simulink model "SerialMonitor_withPRBS"  (R2016b)
settings: Solver=FixedStepDiscrete  StartTime=0.0  StopTime=inf  FixedStep=.01  RelTol=1e-3  EnableMultiTasking=on
StartFcn:
  | s_2 = serial(Port,'BaudRate',115200,'FlowControl','none','Parity','none','DataBits',8,'StopBits',1,'Timeout',2);
  | s_2.InputBufferSize=1024*5; s_2.OutputBufferSize=1024*5;
  | s_2.Terminator='CR';
  | 
  | fopen(s_2);
StopFcn:
  | fclose(s_2);
undefined symbols (not defined in the file or in its folder): serialRead, serialWriteLightBox
libraries: simulink x36, sldrtlib x1
settings Model: Creator=EliteBook 8470p  LastModifiedBy=rsjoshi1
settings DataIOCC: LimitDataPoints=on  SaveFormat=Array
settings OptimizationCC: LifeSpan=inf
settings DebuggingCC: SolverPrmCheckMsg=warning  SFUnexpectedBacktrackingDiag=warning  SFNoUnconditionalDefaultTransitionDiag=warning  SFExecutionAtInitializationDiag=none
settings HardwareCC: ProdBitPerPointer=32  ProdBitPerSizeT=32  ProdBitPerPtrDiffT=32  ProdLargestAtomicFloat=None  ProdIntDivRoundTo=Undefined  ProdEndianess=Unspecified  ProdWordSize=32  ProdHWDeviceType=32-bit Generic
settings ModelReferenceCC: PropagateSignalLabelsOutOfModel=off
settings GRTTargetCC: TargetLangStandard=C89/C90 (ANSI)  GeneratePreprocessorConditionals=Disable all
settings ConfigComp: CovMetricSettings=dw  CovHtmlReporting=on  CovSaveCumulativeToWorkspaceVar=on  CovSaveSingleToWorkspaceVar=on  CovExternalEMLEnable=off  CovSFcnEnable=off

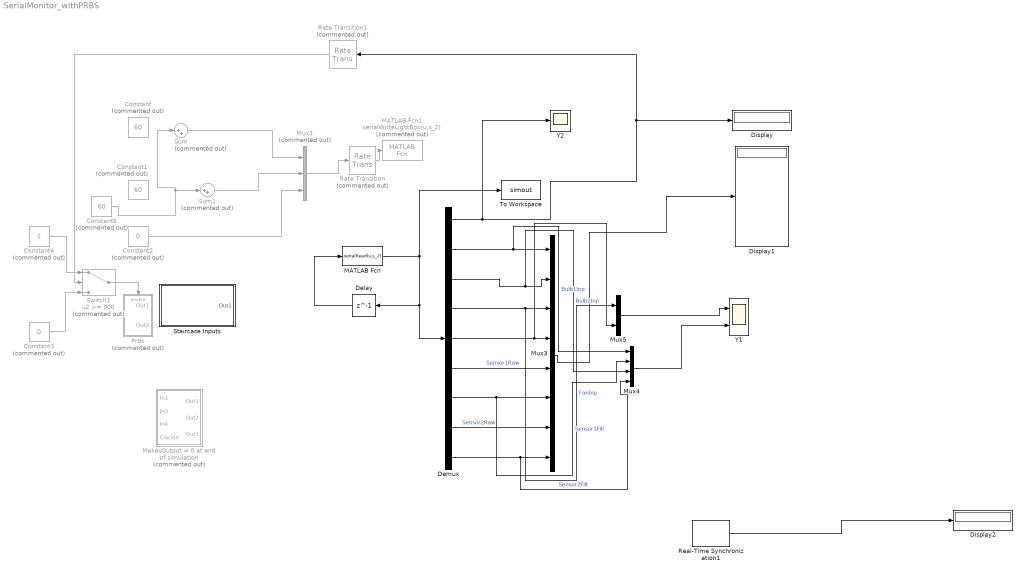
== system SerialMonitor_withPRBS ==
  Constant : Constant  Commented=on  Value=60  OutDataTypeStr=double  SampleTime=0.1
  Constant1 : Constant  Commented=on  Value=60  OutDataTypeStr=double  SampleTime=0.1
  Constant2 : Constant  Commented=on  Value=0  OutDataTypeStr=double  SampleTime=0.1
  Constant3 : Constant  Commented=on  Value=0  SampleTime=0.1
  Constant4 : Constant  Commented=on  SampleTime=0.1
  Constant6 : Constant  Commented=on  Value=60  OutDataTypeStr=double  SampleTime=0.1
  Delay : Delay  DelayLength=1  InitialCondition=0  SampleTime=1
  Demux : Demux  Outputs=9
  Display : Display
  Display1 : Display
  Display2 : Display
  MATLAB Fcn : MATLABFcn  MATLABFcn=serialRead(u,s_2)  OutputDimensions=9
  MATLAB Fcn1 : MATLABFcn  Commented=on  MATLABFcn=serialWriteLightBox(u,s_2)  OutputDimensions=0
  MakesOutput = 0 at end of simulation : Subsystem  Commented=on
  Mux1 : Mux  Commented=on  Inputs=3
  Mux3 : Mux  Inputs=8
  Mux4 : Mux
  Mux5 : Mux  Inputs=2
  Prbs : Subsystem  Commented=on
  Rate Transition : RateTransition  Commented=on  Deterministic=off  OutPortSampleTime=1
  Rate Transition1 : RateTransition  Commented=on  OutPortSampleTime=0.1
  Real-Time Synchronization1 : sldrtlib/Real-Time Synchronization  SampleTime=0.1  MaxMissedTicks=5000  ShowMissedTicks=on  YieldWhenWaiting=off
  Staircase Inputs : Subsystem
  Sum : Sum  Commented=on  Inputs=|++
  Sum1 : Sum  Commented=on  Inputs=|++
  Switch1 : Switch  Commented=on  Threshold=900  SampleTime=0.1
  To Workspace : ToWorkspace  VariableName=simout  SaveFormat=Structure With Time  SampleTime=-1
  Y1 : Scope  NumInputPorts=2
  Y2 : Scope
  wires:
  Delay/1 -> MATLAB Fcn/1
  MATLAB Fcn/1 -> Demux/1, Delay/1, To Workspace/1
  Demux/2 -> Mux4/1, Mux3/1  "Bulb1Inp"
  Demux/3 -> Mux4/3, Mux3/2  "Bulb2Inp"
  Demux/4 -> Mux5/1, Mux3/3  "FanInp"
  Demux/5 -> Mux5/2, Mux3/4
  Demux/6 -> Mux3/5  "Sensor1Raw"
  Demux/7 -> Mux4/2, Mux3/6  "Sensor1Filt"
  Demux/8 -> Mux3/7  "Sensor2Raw"
  Mux1/1 -> Rate Transition/1
  Rate Transition/1 -> MATLAB Fcn1/1
  Real-Time Synchronization1/1 -> Display2/1
  Mux3/1 -> Display1/1
  Constant3/1 -> Switch1/3
  Constant4/1 -> Switch1/1
  Switch1/1 -> Prbs/Enable
  Demux/1 -> Y2/1, Rate Transition1/1, Display/1
  Sum1/1 -> Mux1/2
  Sum/1 -> Mux1/1
  Constant2/1 -> Mux1/3
  Rate Transition1/1 -> Switch1/2
  Demux/9 -> Mux4/4, Mux3/8  "Sensor2Filt"
  Mux4/1 -> Y1/2
  Mux5/1 -> Y1/1
  Constant6/1 -> Sum/1, Sum1/1

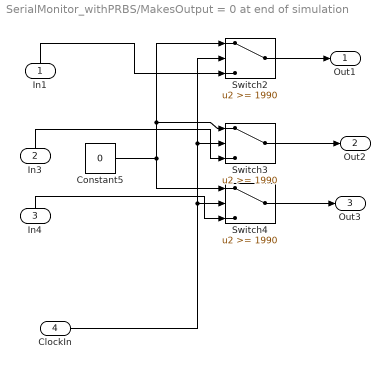
== system SerialMonitor_withPRBS/MakesOutput = 0 at end of simulation ==
  In1 : Inport
  In3 : Inport  Port=2
  In4 : Inport  Port=3
  ClockIn : Inport  Port=4
  Constant5 : Constant  Value=0  SampleTime=0.1
  Switch2 : Switch  Threshold=1990  SampleTime=0.1
  Switch3 : Switch  Threshold=1990  SampleTime=0.1
  Switch4 : Switch  Threshold=1990  SampleTime=0.1
  Out1 : Outport
  Out2 : Outport  Port=2
  Out3 : Outport  Port=3
  wires:
  Switch2/1 -> Out1/1
  ClockIn/1 -> Switch2/2, Switch3/2, Switch4/2
  In1/1 -> Switch2/3
  Switch3/1 -> Out2/1
  In4/1 -> Switch4/3
  Switch4/1 -> Out3/1
  In3/1 -> Switch3/3
  Constant5/1 -> Switch4/1, Switch2/1, Switch3/1

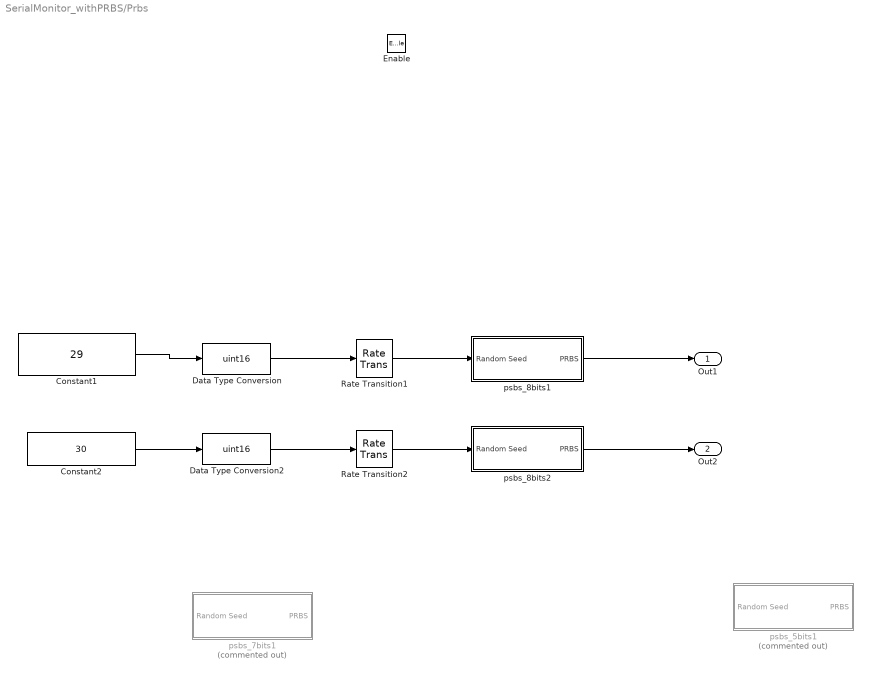
== system SerialMonitor_withPRBS/Prbs ==
  Enable : EnablePort
  Constant1 : Constant  Value=29  OutDataTypeStr=double  SampleTime=0.1
  Constant2 : Constant  Value=30  OutDataTypeStr=double  SampleTime=0.1
  Data Type Conversion : DataTypeConversion  OutDataTypeStr=uint16
  Data Type Conversion2 : DataTypeConversion  OutDataTypeStr=uint16
  Rate Transition1 : RateTransition  OutPortSampleTime=0.1
  Rate Transition2 : RateTransition  OutPortSampleTime=0.1
  psbs_5bits1 : Subsystem  Commented=on  mask(PRBS with 8 shift registers){T=0.1, Tsw=60, Lz=10, Lv=300, Nc=1}
      mask prompts: T "Sample Time (s)"; Tsw "Time to switch (s)"; Lz "Leading Zeros (s)"; Lv "Switching Levels"; Nc "Number of Cycles"
      mask help:
      | Creates a PRBS signal using 6 shift registers.
      |     *Time to switch (Tsw) must be an integer multiple of Sample Time (T).
      |     *Leading zeros specify how long the PRBS will be zero, in seconds, before the levels begin shifting.
      |     *Level is the amplitude of the desired PRBS signal. Both + and - levels are equal
      |     *Number of cycles determines the number of full cycles generated. Each cycle is (2^6-1)*Tsw seconds long
  psbs_7bits1 : Subsystem  Commented=on  mask(PRBS with 8 shift registers){T=0.1, Tsw=60, Lz=10, Lv=300, Nc=1}
      mask prompts: T "Sample Time (s)"; Tsw "Time to switch (s)"; Lz "Leading Zeros (s)"; Lv "Switching Levels"; Nc "Number of Cycles"
      mask help:
      | Creates a PRBS signal using 7 shift registers.
      |     *Time to switch (Tsw) must be an integer multiple of Sample Time (T).
      |     *Leading zeros specify how long the PRBS will be zero, in seconds, before the levels begin shifting.
      |     *Level is the amplitude of the desired PRBS signal. Both + and - levels are equal
      |     *Number of cycles determines the number of full cycles generated. Each cycle is (2^7-1)*Tsw seconds long
  psbs_8bits1 : Subsystem  mask(PRBS with 8 shift registers){T=0.1, Tsw=20, Lz=50, Lv=300, Nc=1}
      mask prompts: T "Sample Time (s)"; Tsw "Time to switch (s)"; Lz "Leading Zeros (s)"; Lv "Switching Levels"; Nc "Number of Cycles"
      mask help:
      | Creates a PRBS signal using 8 shift registers.
      |     *Time to switch (Tsw) must be an integer multiple of Sample Time (T).
      |     *Leading zeros specify how long the PRBS will be zero, in seconds, before the levels begin shifting.
      |     *Level is the amplitude of the desired PRBS signal. Both + and - levels are equal
      |     *Number of cycles determines the number of full cycles generated. Each cycle is (2^8-1)*Tsw seconds long
  psbs_8bits2 : Subsystem  mask(PRBS with 8 shift registers){T=0.1, Tsw=20, Lz=50, Lv=300, Nc=1}
      mask prompts: T "Sample Time (s)"; Tsw "Time to switch (s)"; Lz "Leading Zeros (s)"; Lv "Switching Levels"; Nc "Number of Cycles"
      mask help:
      | Creates a PRBS signal using 8 shift registers.
      |     *Time to switch (Tsw) must be an integer multiple of Sample Time (T).
      |     *Leading zeros specify how long the PRBS will be zero, in seconds, before the levels begin shifting.
      |     *Level is the amplitude of the desired PRBS signal. Both + and - levels are equal
      |     *Number of cycles determines the number of full cycles generated. Each cycle is (2^8-1)*Tsw seconds long
  Out1 : Outport
  Out2 : Outport  Port=2
  wires:
  Constant1/1 -> Data Type Conversion/1
  Data Type Conversion/1 -> Rate Transition1/1
  psbs_8bits1/1(PRBS) -> Out1/1
  Rate Transition1/1 -> psbs_8bits1/1(Random Seed)
  psbs_8bits2/1(PRBS) -> Out2/1
  Rate Transition2/1 -> psbs_8bits2/1(Random Seed)
  Constant2/1 -> Data Type Conversion2/1
  Data Type Conversion2/1 -> Rate Transition2/1

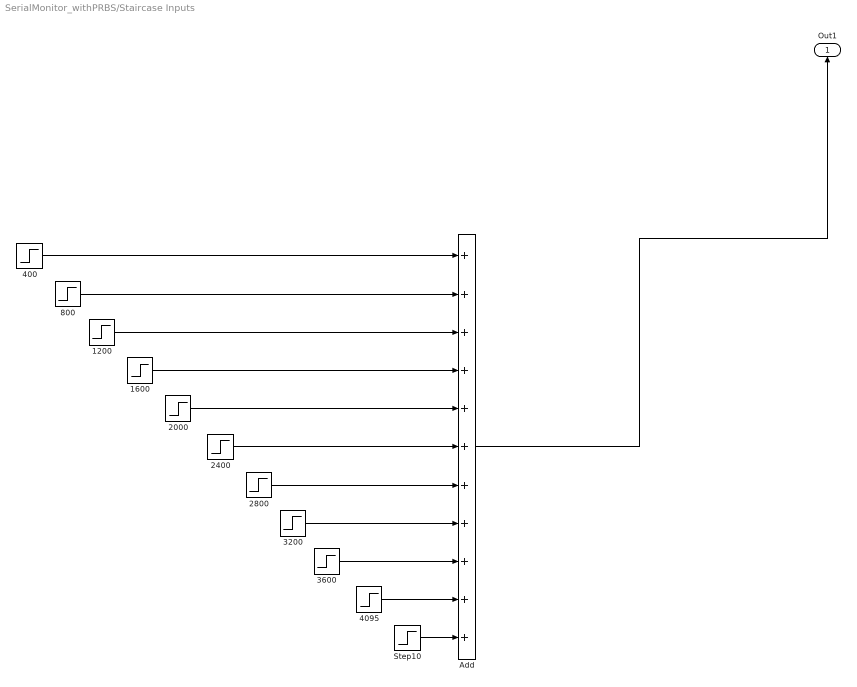
== system SerialMonitor_withPRBS/Staircase Inputs ==
  1200 : Step  Time=70*60  After=400  SampleTime=0.1
  1600 : Step  Time=100*60  After=400  SampleTime=0.1
  2000 : Step  Time=130*60  After=400  SampleTime=0.1
  2400 : Step  Time=160*60  After=400  SampleTime=0.1
  2800 : Step  Time=190*60  After=400  SampleTime=0.1
  3200 : Step  Time=220*60  After=400  SampleTime=0.1
  3600 : Step  Time=250*60  After=400  SampleTime=0.1
  400 : Step  Time=100  After=400  SampleTime=0.1
  4095 : Step  Time=280*60  After=495  SampleTime=0.1
  800 : Step  Time=40*60  After=400  SampleTime=0.1
  Add : Sum  Inputs=+++++++++++
  Step10 : Step  Time=310*60  After=-4095  SampleTime=0.1
  Out1 : Outport
  wires:
  Step10/1 -> Add/11
  3600/1 -> Add/9
  2400/1 -> Add/6
  1200/1 -> Add/3
  3200/1 -> Add/8
  800/1 -> Add/2
  2000/1 -> Add/5
  400/1 -> Add/1
  2800/1 -> Add/7
  1600/1 -> Add/4
  4095/1 -> Add/10
  Add/1 -> Out1/1

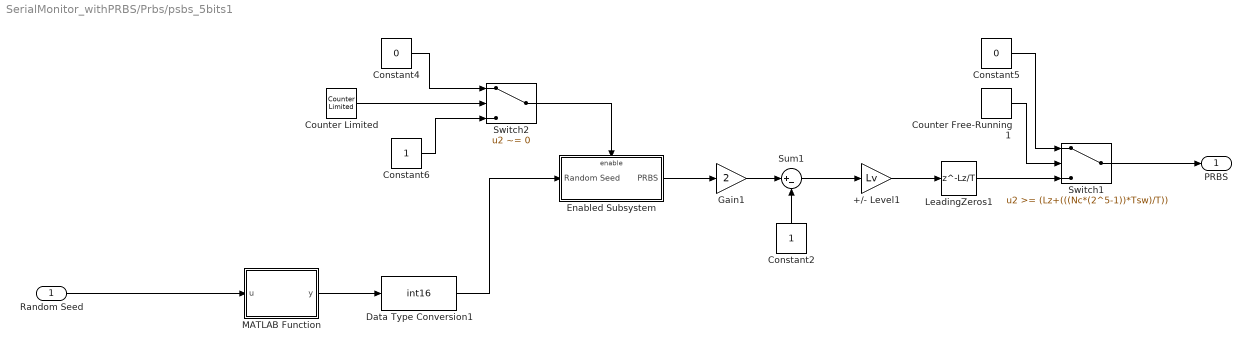
== system SerialMonitor_withPRBS/Prbs/psbs_5bits1 ==
  Random Seed : Inport  OutDataTypeStr=uint16
  +/- Level1 : Gain  Gain=Lv  SampleTime=T
  Constant2 : Constant  SampleTime=T
  Constant4 : Constant  Value=0  SampleTime=T
  Constant5 : Constant  Value=0  SampleTime=T
  Constant6 : Constant  SampleTime=T
  Counter Free-Running1 : simulink/Sources/Counter Free-Running  NumBits=32  tsamp=T
  Counter Limited : simulink/Sources/Counter Limited  uplimit=Tsw/T-1  tsamp=T
  Data Type Conversion1 : DataTypeConversion  OutDataTypeStr=int16
  Enabled Subsystem : Subsystem  TreatAsAtomicUnit=on
  Gain1 : Gain  Gain=2  SampleTime=T
  LeadingZeros1 : Delay  DelayLength=Lz/T  InitialCondition=0  SampleTime=T
  MATLAB Function : MATLAB Function  TreatAsAtomicUnit=on
  Sum1 : Sum  Inputs=|+-  SampleTime=T
  Switch1 : Switch  Threshold=(Lz+(((Nc*(2^5-1))*Tsw)/T))  SampleTime=T
  Switch2 : Switch  Criteria=u2 ~= 0  Threshold=Tsw/T  SampleTime=T
  PRBS : Outport
  wires:
  Counter Limited/1 -> Switch2/2
  Switch2/1 -> Enabled Subsystem/Enable
  Constant4/1 -> Switch2/1
  Constant6/1 -> Switch2/3
  Data Type Conversion1/1 -> Enabled Subsystem/1(Random Seed)
  Enabled Subsystem/1(PRBS) -> Gain1/1
  Sum1/1 -> +/- Level1/1
  Gain1/1 -> Sum1/1
  Constant2/1 -> Sum1/2
  Counter Free-Running1/1 -> Switch1/2
  +/- Level1/1 -> LeadingZeros1/1
  Constant5/1 -> Switch1/1
  LeadingZeros1/1 -> Switch1/3
  MATLAB Function/1(y) -> Data Type Conversion1/1
  Random Seed/1 -> MATLAB Function/1(u)
  Switch1/1 -> PRBS/1

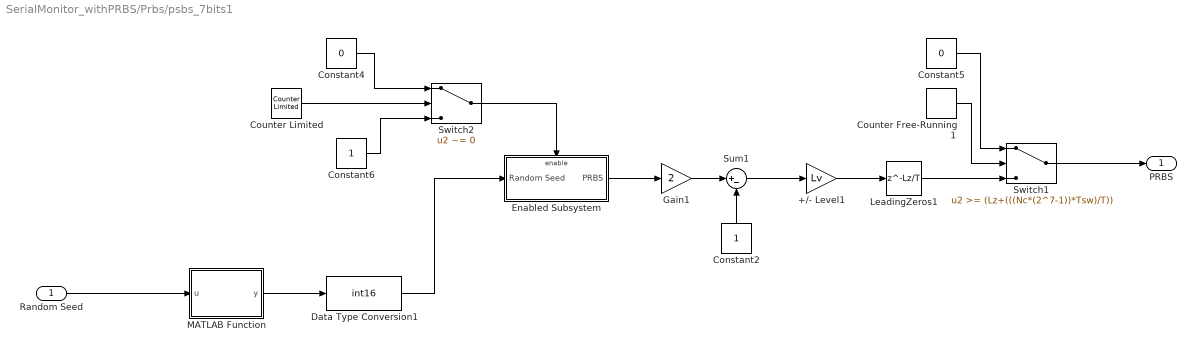
== system SerialMonitor_withPRBS/Prbs/psbs_7bits1 ==
  Random Seed : Inport  OutDataTypeStr=uint16
  +/- Level1 : Gain  Gain=Lv  SampleTime=T
  Constant2 : Constant  SampleTime=T
  Constant4 : Constant  Value=0  SampleTime=T
  Constant5 : Constant  Value=0  SampleTime=T
  Constant6 : Constant  SampleTime=T
  Counter Free-Running1 : simulink/Sources/Counter Free-Running  NumBits=32  tsamp=T
  Counter Limited : simulink/Sources/Counter Limited  uplimit=Tsw/T-1  tsamp=T
  Data Type Conversion1 : DataTypeConversion  OutDataTypeStr=int16
  Enabled Subsystem : Subsystem  TreatAsAtomicUnit=on
  Gain1 : Gain  Gain=2  SampleTime=T
  LeadingZeros1 : Delay  DelayLength=Lz/T  InitialCondition=0  SampleTime=T
  MATLAB Function : MATLAB Function  TreatAsAtomicUnit=on
  Sum1 : Sum  Inputs=|+-  SampleTime=T
  Switch1 : Switch  Threshold=(Lz+(((Nc*(2^7-1))*Tsw)/T))  SampleTime=T
  Switch2 : Switch  Criteria=u2 ~= 0  Threshold=Tsw/T  SampleTime=T
  PRBS : Outport
  wires:
  Switch1/1 -> PRBS/1
  Random Seed/1 -> MATLAB Function/1(u)
  MATLAB Function/1(y) -> Data Type Conversion1/1
  LeadingZeros1/1 -> Switch1/3
  Constant5/1 -> Switch1/1
  +/- Level1/1 -> LeadingZeros1/1
  Counter Free-Running1/1 -> Switch1/2
  Constant2/1 -> Sum1/2
  Gain1/1 -> Sum1/1
  Sum1/1 -> +/- Level1/1
  Enabled Subsystem/1(PRBS) -> Gain1/1
  Data Type Conversion1/1 -> Enabled Subsystem/1(Random Seed)
  Constant6/1 -> Switch2/3
  Constant4/1 -> Switch2/1
  Switch2/1 -> Enabled Subsystem/Enable
  Counter Limited/1 -> Switch2/2

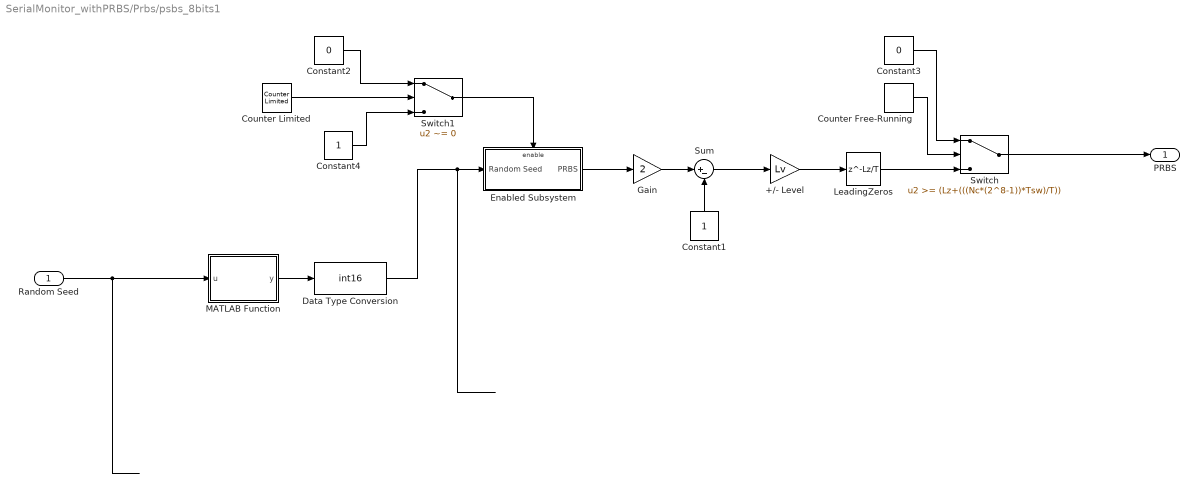
== system SerialMonitor_withPRBS/Prbs/psbs_8bits1 ==
  Random Seed : Inport  OutDataTypeStr=uint16  SampleTime=0.1
  +/- Level : Gain  Gain=Lv  SampleTime=T
  Constant1 : Constant  SampleTime=T
  Constant2 : Constant  Value=0  SampleTime=T
  Constant3 : Constant  Value=0  SampleTime=T
  Constant4 : Constant  SampleTime=T
  Counter Free-Running : simulink/Sources/Counter Free-Running  NumBits=32  tsamp=T
  Counter Limited : simulink/Sources/Counter Limited  uplimit=Tsw/T-1  tsamp=T
  Data Type Conversion : DataTypeConversion  OutDataTypeStr=int16
  Enabled Subsystem : Subsystem  TreatAsAtomicUnit=on
  Gain : Gain  Gain=2  SampleTime=T
  LeadingZeros : Delay  DelayLength=Lz/T  InitialCondition=0  SampleTime=T
  MATLAB Function : MATLAB Function  TreatAsAtomicUnit=on
  Sum : Sum  Inputs=|+-  SampleTime=T
  Switch : Switch  Threshold=(Lz+(((Nc*(2^8-1))*Tsw)/T))  SampleTime=T
  Switch1 : Switch  Criteria=u2 ~= 0  Threshold=Tsw/T  SampleTime=T
  PRBS : Outport
  wires:
  Random Seed/1 -> MATLAB Function/1(u)
  Counter Limited/1 -> Switch1/2
  Switch1/1 -> Enabled Subsystem/Enable
  Constant2/1 -> Switch1/1
  Constant4/1 -> Switch1/3
  Data Type Conversion/1 -> Enabled Subsystem/1(Random Seed)
  Enabled Subsystem/1(PRBS) -> Gain/1
  Sum/1 -> +/- Level/1
  Gain/1 -> Sum/1
  Constant1/1 -> Sum/2
  Counter Free-Running/1 -> Switch/2
  +/- Level/1 -> LeadingZeros/1
  Constant3/1 -> Switch/1
  LeadingZeros/1 -> Switch/3
  MATLAB Function/1(y) -> Data Type Conversion/1
  Switch/1 -> PRBS/1

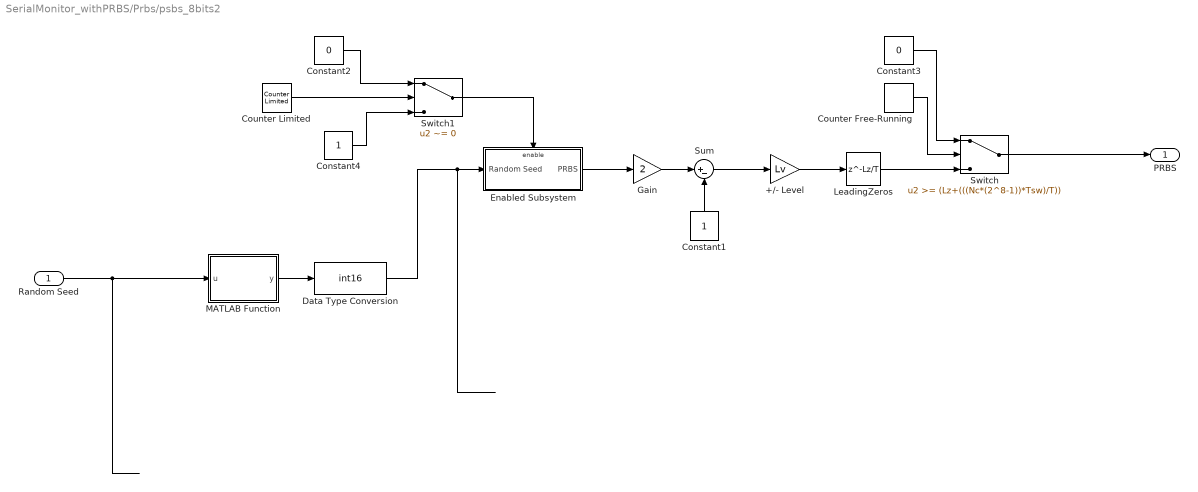
== system SerialMonitor_withPRBS/Prbs/psbs_8bits2 ==
  Random Seed : Inport  OutDataTypeStr=uint16  SampleTime=0.1
  +/- Level : Gain  Gain=Lv  SampleTime=T
  Constant1 : Constant  SampleTime=T
  Constant2 : Constant  Value=0  SampleTime=T
  Constant3 : Constant  Value=0  SampleTime=T
  Constant4 : Constant  SampleTime=T
  Counter Free-Running : simulink/Sources/Counter Free-Running  NumBits=32  tsamp=T
  Counter Limited : simulink/Sources/Counter Limited  uplimit=Tsw/T-1  tsamp=T
  Data Type Conversion : DataTypeConversion  OutDataTypeStr=int16
  Enabled Subsystem : Subsystem  TreatAsAtomicUnit=on
  Gain : Gain  Gain=2  SampleTime=T
  LeadingZeros : Delay  DelayLength=Lz/T  InitialCondition=0  SampleTime=T
  MATLAB Function : MATLAB Function  TreatAsAtomicUnit=on
  Sum : Sum  Inputs=|+-  SampleTime=T
  Switch : Switch  Threshold=(Lz+(((Nc*(2^8-1))*Tsw)/T))  SampleTime=T
  Switch1 : Switch  Criteria=u2 ~= 0  Threshold=Tsw/T  SampleTime=T
  PRBS : Outport
  wires:
  Switch/1 -> PRBS/1
  MATLAB Function/1(y) -> Data Type Conversion/1
  LeadingZeros/1 -> Switch/3
  Constant3/1 -> Switch/1
  +/- Level/1 -> LeadingZeros/1
  Counter Free-Running/1 -> Switch/2
  Constant1/1 -> Sum/2
  Gain/1 -> Sum/1
  Sum/1 -> +/- Level/1
  Enabled Subsystem/1(PRBS) -> Gain/1
  Data Type Conversion/1 -> Enabled Subsystem/1(Random Seed)
  Constant4/1 -> Switch1/3
  Constant2/1 -> Switch1/1
  Switch1/1 -> Enabled Subsystem/Enable
  Counter Limited/1 -> Switch1/2
  Random Seed/1 -> MATLAB Function/1(u)

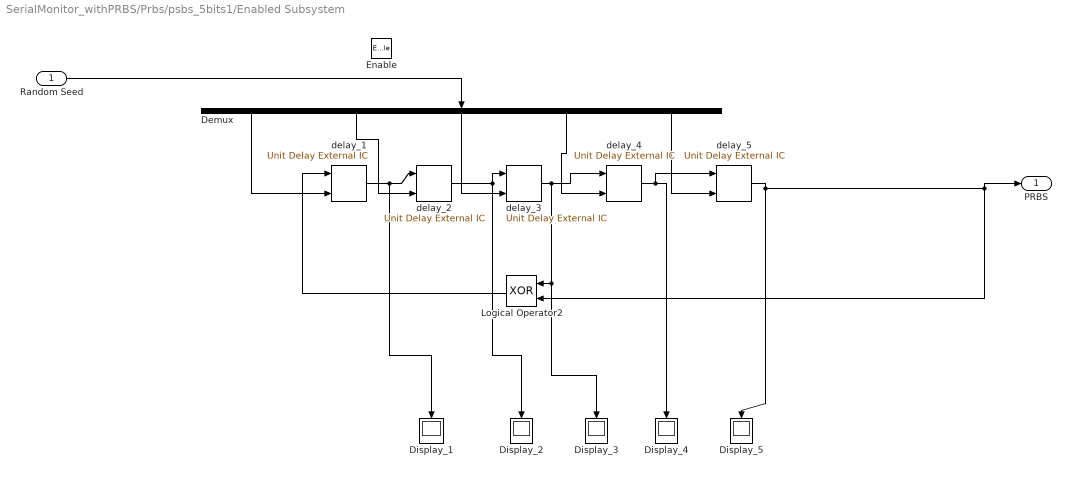
== system SerialMonitor_withPRBS/Prbs/psbs_5bits1/Enabled Subsystem ==
  Random Seed : Inport  OutDataTypeStr=int16
  Enable : EnablePort
  Demux : Demux  Outputs=5
  Display_{1..5} (5 alike) : Display
  Logical Operator2 : Logic  Operator=XOR  AllPortsSameDT=off  OutDataTypeStr=fixdt(1,16)  SampleTime=T
  delay_{1..5} (5 alike) : simulink/Additional Math & Discrete/Additional Discrete/Unit Delay External IC  tsamp=T
  PRBS : Outport
  wires:
  Random Seed/1 -> Demux/1
  delay_5/1 -> Logical Operator2/2, PRBS/1, Display_5/1
  Logical Operator2/1 -> delay_1/1
  Demux/1 -> delay_1/2
  Demux/2 -> delay_2/2
  Demux/3 -> delay_3/2
  Demux/4 -> delay_4/2
  Demux/5 -> delay_5/2
  delay_1/1 -> Display_1/1, delay_2/1
  delay_4/1 -> Display_4/1, delay_5/1
  delay_3/1 -> delay_4/1, Logical Operator2/1, Display_3/1
  delay_2/1 -> delay_3/1, Display_2/1

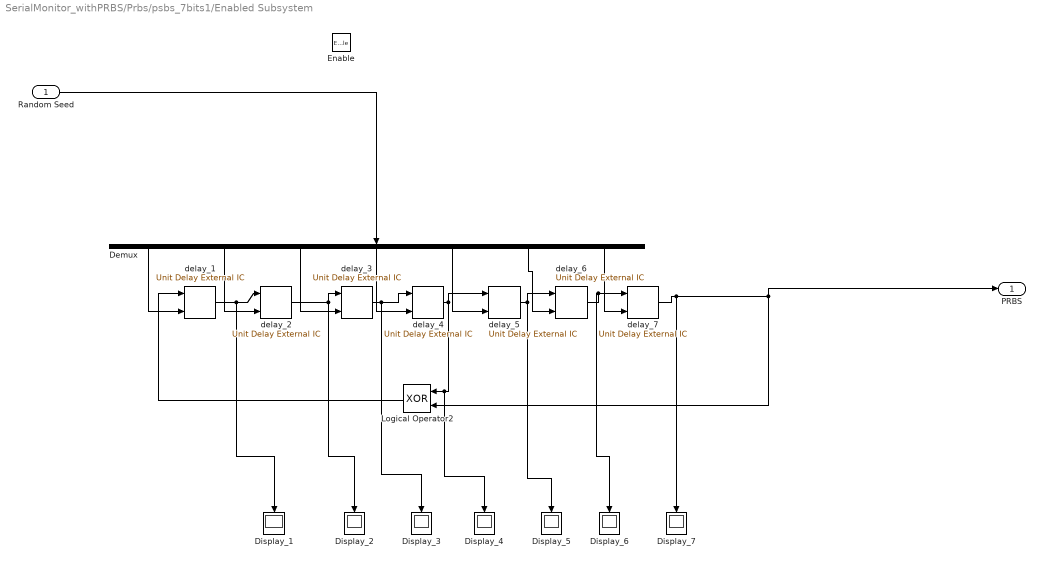
== system SerialMonitor_withPRBS/Prbs/psbs_7bits1/Enabled Subsystem ==
  Random Seed : Inport  OutDataTypeStr=int16
  Enable : EnablePort
  Demux : Demux  Outputs=7
  Display_{1..7} (7 alike) : Display
  Logical Operator2 : Logic  Operator=XOR  AllPortsSameDT=off  OutDataTypeStr=fixdt(1,16)  SampleTime=T
  delay_{1..7} (7 alike) : simulink/Additional Math & Discrete/Additional Discrete/Unit Delay External IC  tsamp=T
  PRBS : Outport
  wires:
  delay_7/1 -> Logical Operator2/2, PRBS/1, Display_7/1
  delay_5/1 -> Display_5/1, delay_6/1
  delay_6/1 -> Display_6/1, delay_7/1
  delay_2/1 -> Display_2/1, delay_3/1
  delay_3/1 -> Display_3/1, delay_4/1
  delay_4/1 -> Display_4/1, Logical Operator2/1, delay_5/1
  delay_1/1 -> delay_2/1, Display_1/1
  Demux/7 -> delay_7/2
  Demux/6 -> delay_6/2
  Demux/5 -> delay_5/2
  Demux/4 -> delay_4/2
  Demux/3 -> delay_3/2
  Demux/2 -> delay_2/2
  Demux/1 -> delay_1/2
  Random Seed/1 -> Demux/1
  Logical Operator2/1 -> delay_1/1

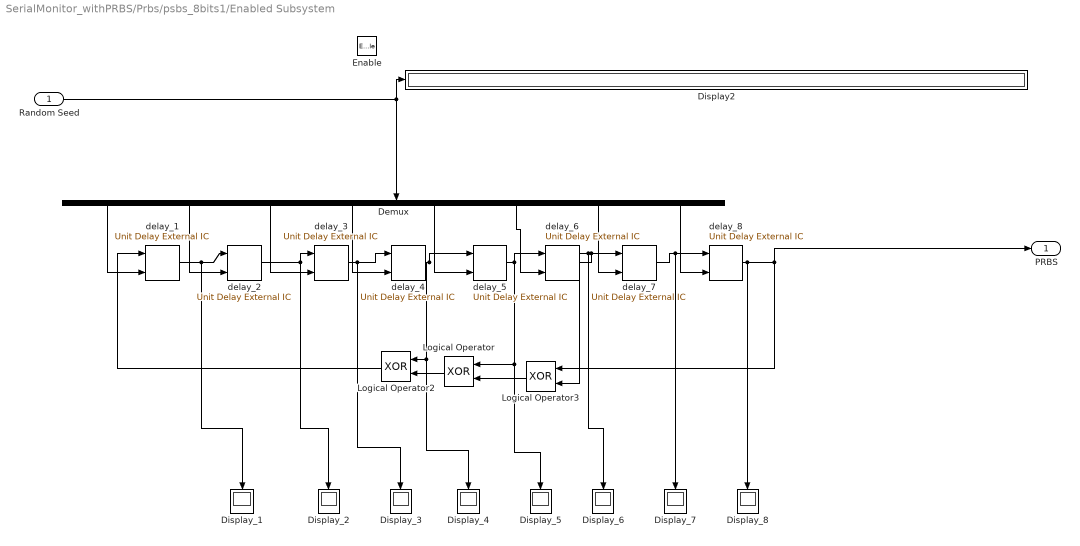
== system SerialMonitor_withPRBS/Prbs/psbs_8bits1/Enabled Subsystem ==
  Random Seed : Inport  OutDataTypeStr=int16
  Enable : EnablePort
  Demux : Demux  Outputs=8
  Display2 : Display
  Display_{1..8} (8 alike) : Display
  Logical Operator : Logic  Operator=XOR  AllPortsSameDT=off  OutDataTypeStr=fixdt(1,16)  SampleTime=T
  Logical Operator2 : Logic  Operator=XOR  AllPortsSameDT=off  OutDataTypeStr=fixdt(1,16)  SampleTime=T
  Logical Operator3 : Logic  Operator=XOR  AllPortsSameDT=off  OutDataTypeStr=fixdt(1,16)  SampleTime=T
  delay_{1..8} (8 alike) : simulink/Additional Math & Discrete/Additional Discrete/Unit Delay External IC  tsamp=T
  PRBS : Outport
  wires:
  delay_5/1 -> Display_5/1, Logical Operator/1, delay_6/1
  delay_6/1 -> Logical Operator3/2, Display_6/1, delay_7/1
  delay_2/1 -> Display_2/1, delay_3/1
  delay_3/1 -> Display_3/1, delay_4/1
  delay_4/1 -> Display_4/1, Logical Operator2/1, delay_5/1
  delay_1/1 -> delay_2/1, Display_1/1
  delay_7/1 -> Display_7/1, delay_8/1
  Logical Operator/1 -> Logical Operator2/2
  Logical Operator3/1 -> Logical Operator/2
  Random Seed/1 -> Display2/1, Demux/1
  Demux/8 -> delay_8/2
  Demux/7 -> delay_7/2
  Demux/6 -> delay_6/2
  Demux/5 -> delay_5/2
  Demux/4 -> delay_4/2
  Demux/3 -> delay_3/2
  Demux/2 -> delay_2/2
  Demux/1 -> delay_1/2
  Logical Operator2/1 -> delay_1/1
  delay_8/1 -> Logical Operator3/1, PRBS/1, Display_8/1

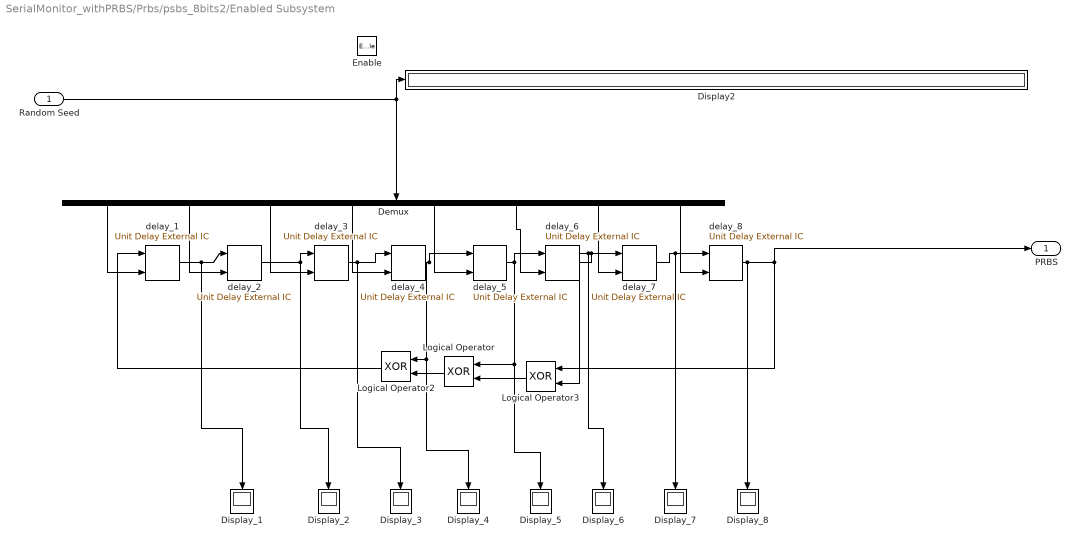
== system SerialMonitor_withPRBS/Prbs/psbs_8bits2/Enabled Subsystem ==
  Random Seed : Inport  OutDataTypeStr=int16
  Enable : EnablePort
  Demux : Demux  Outputs=8
  Display2 : Display
  Display_{1..8} (8 alike) : Display
  Logical Operator : Logic  Operator=XOR  AllPortsSameDT=off  OutDataTypeStr=fixdt(1,16)  SampleTime=T
  Logical Operator2 : Logic  Operator=XOR  AllPortsSameDT=off  OutDataTypeStr=fixdt(1,16)  SampleTime=T
  Logical Operator3 : Logic  Operator=XOR  AllPortsSameDT=off  OutDataTypeStr=fixdt(1,16)  SampleTime=T
  delay_{1..8} (8 alike) : simulink/Additional Math & Discrete/Additional Discrete/Unit Delay External IC  tsamp=T
  PRBS : Outport
  wires:
  delay_8/1 -> Display_8/1, PRBS/1, Logical Operator3/1
  Logical Operator2/1 -> delay_1/1
  Demux/1 -> delay_1/2
  Demux/2 -> delay_2/2
  Demux/3 -> delay_3/2
  Demux/4 -> delay_4/2
  Demux/5 -> delay_5/2
  Demux/6 -> delay_6/2
  Demux/7 -> delay_7/2
  Demux/8 -> delay_8/2
  Random Seed/1 -> Demux/1, Display2/1
  Logical Operator3/1 -> Logical Operator/2
  Logical Operator/1 -> Logical Operator2/2
  delay_7/1 -> delay_8/1, Display_7/1
  delay_1/1 -> Display_1/1, delay_2/1
  delay_4/1 -> delay_5/1, Logical Operator2/1, Display_4/1
  delay_3/1 -> delay_4/1, Display_3/1
  delay_2/1 -> delay_3/1, Display_2/1
  delay_6/1 -> delay_7/1, Display_6/1, Logical Operator3/2
  delay_5/1 -> delay_6/1, Logical Operator/1, Display_5/1

== matlab function SerialMonitor_withPRBS/Prbs/psbs_8bits1/MATLAB Function ==
  data: u input; y output
function y = fcn(u)
%#codegen
y = zeros(8,1);
% s = de2bi(u,16);
s = dec2bin(u,16);
y(1) = s(end-7)-48;
y(2) = s(end-6)-48;
y(3) = s(end-5)-48;
y(4) = s(end-4)-48;
y(5) = s(end-3)-48;
y(6) = s(end-2)-48;
y(7) = s(end-1)-48;
y(8) = s(end)-48;

== matlab function SerialMonitor_withPRBS/Prbs/psbs_7bits1/MATLAB Function ==
  data: u input; y output
function y = fcn(u)
%#codegen
y = zeros(7,1);
% s = de2bi(u,16);
s = dec2bin(u,16);
y(1) = s(end-6)-48;
y(2) = s(end-5)-48;
y(3) = s(end-4)-48;
y(4) = s(end-3)-48;
y(5) = s(end-2)-48;
y(6) = s(end-1)-48;
y(7) = s(end)-48;

== matlab function SerialMonitor_withPRBS/Prbs/psbs_5bits1/MATLAB Function ==
  data: u input; y output
function y = fcn(u)
%#codegen
y = zeros(5,1);
% s = de2bi(u,16);
s = dec2bin(u,16);
y(1) = s(end-4)-48;
y(2) = s(end-3)-48;
y(3) = s(end-2)-48;
y(4) = s(end-1)-48;
y(5) = s(end)-48;

== matlab function SerialMonitor_withPRBS/Prbs/psbs_8bits2/MATLAB Function ==
  data: u input; y output
function y = fcn(u)
%#codegen
y = zeros(8,1);
% s = de2bi(u,16);
s = dec2bin(u,16);
y(1) = s(end-7)-48;
y(2) = s(end-6)-48;
y(3) = s(end-5)-48;
y(4) = s(end-4)-48;
y(5) = s(end-3)-48;
y(6) = s(end-2)-48;
y(7) = s(end-1)-48;
y(8) = s(end)-48;
